simulink subsystem "LVSS_EN"  (R2023b)
settings: Solver=VariableStepAuto  StartTime=0.0  StopTime=50  RelTol=1e-3
settings Model: DefaultTestHarness=LVSS_EN_Harness1  Creator=diego  LastModifiedBy=heyka

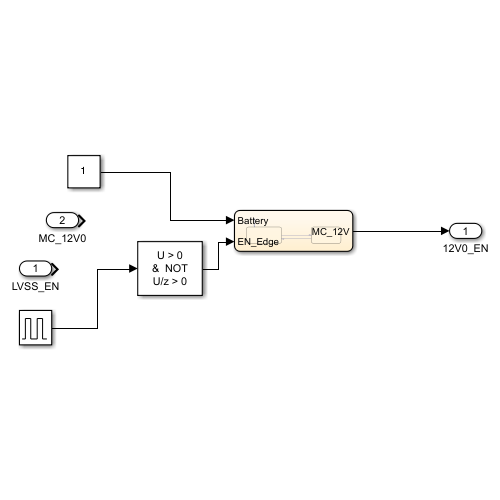
[thumbnail: Simulink's stored preview of the top-level diagram]
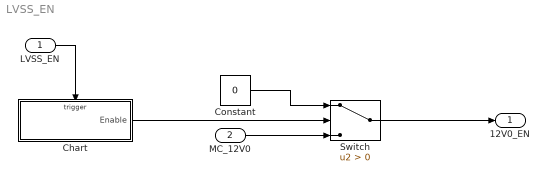
== system LVSS_EN ==
  LVSS_EN : Inport
  MC_12V0 : Inport  Port=2
  Chart : Stateflow chart  TreatAsAtomicUnit=on
  Constant : Constant  Value=0
  Switch : Switch  Criteria=u2 > Threshold  SaturateOnIntegerOverflow=off  InputSameDT=off
  12V0_EN : Outport
  wires:
  Switch/1 -> 12V0_EN/1
  LVSS_EN/1 -> Chart/Trigger
  Chart/1(Enable) -> Switch/2
  MC_12V0/1 -> Switch/3
  Constant/1 -> Switch/1

== stateflow chart LVSS_EN/Chart ==
  settings: executeAtInitialization=1
  state Off
    entry:
    Enable = 0;
  state On1
    entry:
    Enable = 1;
  (default) -> On1
  Off -> On1 : Transition
  On1 -> Off : Transition
  data: Enable output =0
  events: Transition input RISING_EDGE_EVENT
